simulink model "Force_Att_Controller_Separated"  (R2020a)
settings: Solver=FixedStepAuto  StartTime=0.0  StopTime=20  FixedStep=P.Ts  RelTol=1e-3
PreLoadFcn:
  | parameters
values from neighbouring files (symbols this model uses):
  beta1 = 1    [Run_force_Att_Controller.m]
  kTheta = 0.5/N    (= 0.00333333333333)    [Run_force_Att_Controller.m]
  L = 3    [Run_force_Att_Controller.m]
  m = 3    [Run_force_Att_Controller.m]
  n = length(q)    [Run_force_Att_Controller.m]    (also in circlePoints.m = numberOfPoints)
  N = 150    [Run_force_Att_Controller.m]
  T1 = 1    [Run_force_Att_Controller.m]
  T2 = 0.6    [Run_force_Att_Controller.m]
  ThetaHat0 = [ones(9,1)*1;1]    [Run_force_Att_Controller.m]
  ThetaStar = [0.2061;0.2061;0.2061;0.2061;0.2061;0.2061;6.7315;2.6926;0;1.5]    [Run_force_Att_Controller.m]
  Ts = P.Ts    [Run_force_Att_Controller.m]
  x1_int = [0;-0.15;0.5]    [Run_force_Att_Controller.m]
  x1Dot = [0;0;0]    [Run_force_Att_Controller.m]
  x2_int = [0;0.15;0.5]    [Run_force_Att_Controller.m]
  x2Dot = [0;0;0]    [Run_force_Att_Controller.m]
  xc_int = [0;0;0.5]    [Run_force_Att_Controller.m]
  xcDot = [0;0;0]    [Run_force_Att_Controller.m]
undefined symbols (not defined in the file or in its folder): P
(part 2 of 2)

== matlab function Force_Att_Controller_Separated/Subsystem/PayloadForceController ==
  data: thetahatdot input; Gamma input; x1 input; x1Dot input; t input; x2 input; x2Dot input; xc input; p input; q input; x1DDot output; des_state1 output; des_thrust1 output; ct_force output; AM output; des_state2 output; des_thrust2 output; x2DDot output; xcDDot output; P parameter; u output; pD output; qD output; thetahatdotNC output; thetahatNC input; f1Star output; ThetaTilde output; ThetaStar parameter
function [x1DDot,des_state1, des_thrust1,ct_force,AM, des_state2, des_thrust2,  x2DDot,  xcDDot,u,pD,qD, thetahatdotNC,f1Star,ThetaTilde]     = PayLoad(thetahatdot,Gamma,x1,x1Dot,t,x2,x2Dot,xc,p,q, P, thetahatNC,ThetaStar)
%% PayLoad Force Controller 
x1 = p(1:3,1);
x2 = p(4:6,1);
xc = p(7:9,1);
x1Dot = q(1:3,1);
x2Dot = q(4:6,1);
xcDot = q(7:9,1);
Theta1Dot_CL = thetahatdot(1:3);
Theta2Dot_CL = thetahatdot(4:6);
theta_cDot_CL = thetahatdot(7:end);
m1 = P.m;
m2 = m1;
Mc = P.Mc;
g = P.g;
k = P.k;

C1x = 0.2061;%0.2 + 0.9*exp(-0.6*norm(-x1Dot) -2); 
C1y = 0.2061;%0.2 + 0.9*exp(-0.6*norm(-x1Dot) -2); 
C1z = 0.2061;%0.2 + 0.9*exp(-0.6*norm(-x1Dot) -2); 
C1 = diag([C1x, C1y, C1z]);

C2x = 0.2061;%0.2 + 0.9*exp(-0.6*norm(-x2Dot) -2); 
C2y = 0.2061;%0.2 + 0.9*exp(-0.6*norm(-x2Dot) -2); 
C2z = 0.2061;%0.2 + 0.9*exp(-0.6*norm(-x2Dot) -2); 
C2 = diag([C2x, C2y, C2z]);
Cc = 0.25;

% Cf_act = [C1x; C1y; C1z; C2x ; C2y ; C2z];

e3 = [0 0 1]';

R_theta = eye(3,3);     
% xc = [0;0;0.5];
r1 = [0 -0.15 0]';
r2 = [0 0.15 0]';

a1 = xc + R_theta*r1; 

a2 = xc + R_theta*r2;

z1 = x1 - a1;

z2 = x2 - a2;

% k = 2.5*10e4;
f1 = k*z1;  % linear model 
% f1 = k*norm(z1)*z1; % second order model
f2 = k*z2;   % linear model 
% f2 = k*norm(z2)*z2;   %second order model

% v1d = (1-exp(-t))*[5.0  2.0 0.0]';
% v2d = (1-exp(-t))*[5.0  2.0 0.0]';

k_cc = (1-exp(-1*t));

%%%%%%%%%%%%%%%%%%%%%%%%%%%%%%%%%%%%%%%%%%%%%%%%%%%%%%%%%%%%%%
% Un comment for time varying velocity 
if t<= 5
    v1d = k_cc*[t 0.4*t 0]';
    v2d = k_cc*[t 0.4*t 0]';
    vdDot = [1 0.4 0]';
elseif t <= 10
    v1d = k_cc*[5 2 0 ]';
    v2d = k_cc*[5 2 0 ]';
    vdDot = [0 0 0]';
elseif t<=15
    v1d = k_cc*[-t+15 -0.4*t+6 0]';
    v2d = k_cc*[-t+15 -0.4*t+6 0]';
    vdDot = [-1 -0.4 0]';
else 
    v1d = [0 0 0]';
    v2d = [0 0 0]';
    vdDot = [0 0 0]';
end 
%%%%%%%%%%%%%%%%%%%%%%%%%%%%%%%%%%%%%%%%%%%%%%%%%%%%%%%%%%%%%%

%%%%%%%%%%%%%%%%%%%%%%%%%%%%%%%%%%%%%%%%%%%%%%%%%%%%%%%%%%%%%%
% Un comment for constant velocity 
% v1d = k_cc*[5.0  2.0 0.0]';
% v2d = k_cc*[5.0  2.0 0.0]';
% vdDot = [0 0 0]';
%%%%%%%%%%%%%%%%%%%%%%%%%%%%%%%%%%%%%%%%%%%%%%%%%%%%%%%%%%%%%%

%%%%%%%%%%%%%%%%%%%%%%%%%%%%%%%%%%%%%%%%%%%%%%%%%%%%%%%%%%%%%%%%%%%
% Leave the below uncommented/just for trail and error

% if t<= 5
%     v1d = k_cc*[t 0.5*t 0]';
%     v2d = k_cc*[t 0.5*t 0]';
% elseif t <= 15
%     v1d = k_cc*[5 2 0 ]';
%     v2d = k_cc*[5 2 0 ]';
% elseif t<=20
%     v1d = k_cc*[-t+20 -0.5*t+10 0]';
%     v2d = k_cc*[-t+20 -0.5*t+10 0]';
% else 
%     v1d = [0 0 0]';
%     v2d = [0 0 0]';
% end 
% 
% if t<= 5
%     v1d = k_cc*[0 0 0 ]';
%     v2d = k_cc*[0 0 0 ]';
% elseif t <= 10 
%     v1d = k_cc*[2 1 0 ]';
%     v2d = k_cc*[2 1 0 ]';
% else 
%     v1d = k_cc*[0 0 0 ]';
%     v2d = k_cc*[0 0 0 ]';
% end 
% v1d = 5-5*exp(-10*t)*[1 0 0]'; 
% v2d = 5-5*exp(-10*t)*[1 0 0]';

% if t < 2
% v1d = [2.0 1.0 0.1]';
% v2d = [2.0 1.0 0.1]';
% else 
%     v1d = [2.0 1.0 0]';
%     v2d = [2.0 1.0 0]';
% end 

% v1d = [0 0 0]';
% v2d = [0 0 0]';
%%%%%%%%%%%%%%%%%%%%%%%%%%%%%%%%%%%%%%%%%%%%%%%%%%%%%%%%%%%%%%%%%%%%

Y_f = [eye(3),g*e3];
N= 2; 

Xi_1 = x1Dot - v1d; 
Xi_2 = x2Dot - v2d; 

sum_Xi = Xi_1 + Xi_2;

Phi1 = [Xi_1(1)*x1Dot(1), Xi_1(2)*x1Dot(2) ,Xi_1(3)*x1Dot(3)];
Phi2 = [Xi_2(1)*x2Dot(1), Xi_2(2)*x2Dot(2) ,Xi_2(3)*x2Dot(3)];

if t <= 1.0
    Gamma = 0.01*eye(10,10); 
    ke = 10e6;

    Theta_cDot = -Gamma(7:10,7:10)/ke*(1/N*Y_f'*sum_Xi) + theta_cDot_CL;
    % Theta_cDot = -0.01*(1/N*Y_f'*sum_Xi) + theta_cDot_CL;
    
    C1Dot = -Gamma(1:3,1:3)/ke*Phi1' + Theta1Dot_CL;
    C2Dot = -Gamma(4:6,4:6)/ke*Phi2' + Theta2Dot_CL;
    
else 
    
    ke = 10e6;
    
    Theta_cDot = -Gamma(7:10,7:10)/ke*(1/N*Y_f'*sum_Xi) + theta_cDot_CL;
    % Theta_cDot = -0.01*(1/N*Y_f'*sum_Xi) + theta_cDot_CL;
    
    C1Dot = -norm(x1Dot)*Gamma(1:3,1:3)/ke*Phi1' + Theta1Dot_CL;
    C2Dot = -norm(x2Dot)*Gamma(4:6,4:6)/ke*Phi2' + Theta2Dot_CL;
    
end

% C1Dot = -0.01*Phi1' + Theta1Dot_CL; 
% C2Dot = -0.01*Phi2' + Theta2Dot_CL; 

thetahatdotNC = [C1Dot; C2Dot; Theta_cDot];

C1Hat = thetahatNC(1:3); 
C2Hat = thetahatNC(4:6); 
Theta_cHat = thetahatNC(7:10);

f1d = k_cc*1/N*Y_f*Theta_cHat ;
f2d = k_cc*1/N*Y_f*Theta_cHat ;

fd = [f1d;f2d];

Ki  = 1*[150 0 0;
          0 150 0;
          0 0  150];

% Ki  = 1*[100 0 0;
%           0 100 0;
%           0 0  100];
% 
F1 = -Ki*(x1Dot - v1d) + f1d  + m1*g*e3+ diag(C1Hat)*norm(x1Dot)*x1Dot + m1*vdDot;
F2 = -Ki*(x2Dot - v2d) + f2d + m2*g*e3+ diag(C2Hat)*norm(x2Dot)*x2Dot +  m2*vdDot; 

T1 = sqrt(F1'*F1);
T2 = sqrt(F2'*F2);

psi1 = 0.0; 
psi2 = 0.0;

% psi1 = 0.0872665;
% psi2 = 0.0872665;

theta1 = atan((F1(1)*cos(psi1) + F1(2)*sin(psi1))/F1(3));
theta2 = atan((F2(1)*cos(psi2) + F2(2)*sin(psi2))/F2(3));

% theta1 = 0.1745; 
% theta2 = 0.1745; 

phi1 = asin((F1(1)*sin(psi1) - F1(2)*cos(psi1))/(T1));
phi2 = asin((F2(1)*sin(psi2) - F2(2)*cos(psi2))/(T2));

% phi1 = 0.1745; 
% phi2 = 0.1745; 

R_b1 = [ cos(psi1)*cos(theta1), cos(psi1)*sin(phi1)*sin(theta1) - cos(phi1)*sin(psi1), sin(phi1)*sin(psi1) + cos(phi1)*cos(psi1)*sin(theta1);
    cos(theta1)*sin(psi1), cos(phi1)*cos(psi1) + sin(phi1)*sin(psi1)*sin(theta1),   cos(phi1)*sin(psi1)*sin(theta1) - cos(psi1)*sin(phi1);
    -sin(theta1),         cos(theta1)*sin(phi1),                              cos(phi1)*cos(theta1)];

R_b2 = [ cos(psi2)*cos(theta2), cos(psi2)*sin(phi2)*sin(theta2) - cos(phi2)*sin(psi2), sin(phi2)*sin(psi2) + cos(phi2)*cos(psi2)*sin(theta2);
    cos(theta2)*sin(psi2), cos(phi2)*cos(psi2) + sin(phi2)*sin(psi2)*sin(theta2),   cos(phi2)*sin(psi2)*sin(theta2) - cos(psi2)*sin(phi2);
    -sin(theta2),         cos(theta2)*sin(phi2),                              cos(phi2)*cos(theta2)];

l1 = [0 -0.2 0.2]';
AM1 = (x1)+ R_b1*l1;
l2 = [0 0.2 0.2]';
AM2 = (x2) + R_b2*l2;

AM = [AM1;AM2];

% e3 = [0 0 1]';
F1d = T1*R_b1*e3;
F2d = T2*R_b2*e3;
%     end
ct_force = [f1];
des_angle1 = [phi1 ;theta1; psi1]; % in the order ZYX [psi1 theta1 phi1] -->> [Zangle Yangle Xangle]
des_state1 = [des_angle1;0;0;0];
des_angle2 = [phi2 ;theta2; psi2]; % 
des_state2 = [des_angle2;0;0;0];
des_thrust1 = T1;
des_thrust2 = T2;
x1DDot = (F1 - f1 -  m1*g*e3 - C1*norm(x1Dot)*x1Dot)/m1; 
x2DDot = (F2 - f2 - m2*g*e3 - C2*norm(x2Dot)*x2Dot)/m2;
% f_z = [0 0 20]';
% F_d = [5.39; 2.15; 0];
F_d = [6.7315;2.6926;0];
% xcDDot = (f1 + f2 - Mc*e3*g - Cc*eye(3)*norm(xcDot)*xcDot )/Mc;
xcDDot = (f1 + f2 - Mc*e3*g - F_d )/Mc;
pD = [q];
qD = [x1DDot;x2DDot;xcDDot];
u = [F1;F2];
ThetaTilde = ThetaStar - thetahatNC;
f1Star = 1/N*Y_f*ThetaStar(7:10,1);
% des_accln1 = x1DDot;
% des_accln2 = x2DDot;
